simulink model "CLRFSPFCRealizedSimscape"  (R2025a)
settings: Solver=daessc  StartTime=0.0  StopTime=tend  FixedStep=tstep  MaxStep=1e-6  RelTol=1e-3  AbsTol=1e-4
undefined symbols (not defined in the file): Cf, fg, ncycles_end, Rc1, Rc2, Rc3, Rclp, Rin1, Rin2, Rin3, Rout, Rst1, Rst2, tend, Vc, Vg
libraries: fl_lib x48, nesl_utility x13, ee_lib x7, simulink x3, eePowerMeasurement x1, eeRmsMeasurement x1
settings Model: Creator=FactCore  LastModifiedBy=FactCore
settings SolverCC: ZeroCrossAlgorithm=Adaptive  SolverResetMethod=Robust
settings DataIOCC: SaveTime=off
settings HardwareCC: ProdHWDeviceType=AMD->x86-64 (Windows64)
settings SFSimCC: SimTargetLang=C++  SimDLTargetLibrary=mkl-dnn

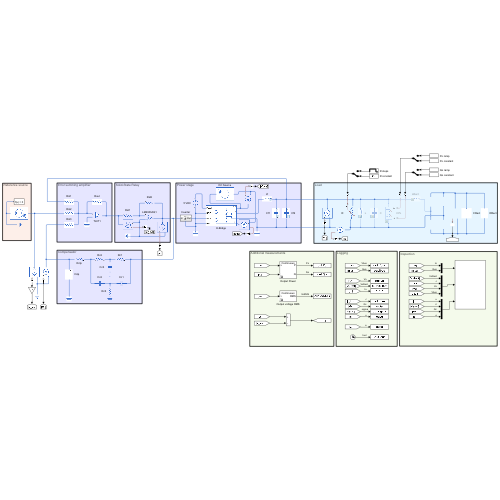
[thumbnail: Simulink's stored preview of the top-level diagram]
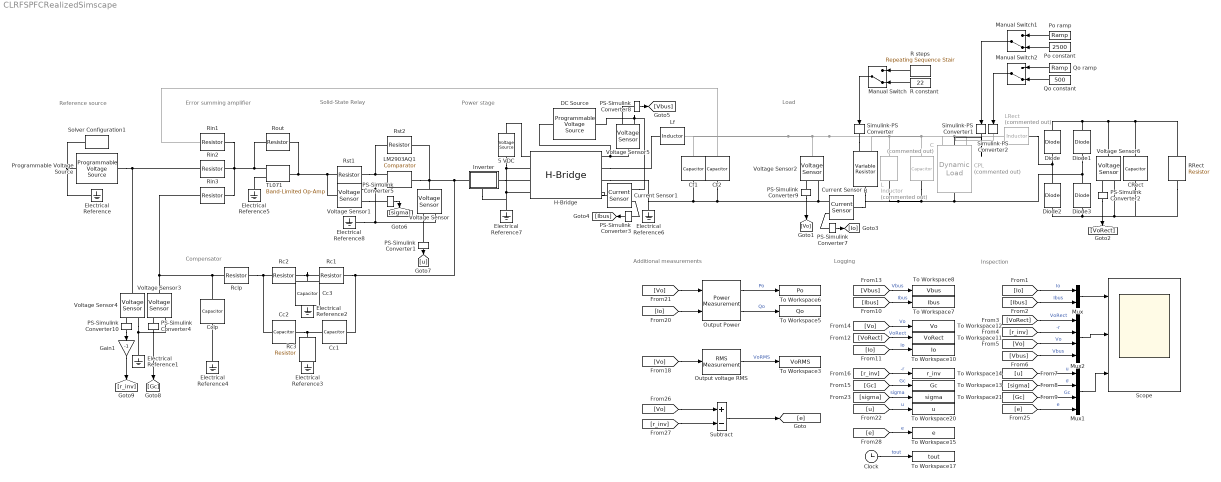
== system CLRFSPFCRealizedSimscape ==
  note: Additional measurements
  note: Inspection
  note: Logging
  note: Reference source
  note: Error summing amplifier
  note: Compensator
  note: Load
  note: Power stage
  note: Solid-State Relay
  5 VDC : ee_lib/Sources/Voltage Source  dc_voltage=5 V  ac_voltage=0 V  ac_shift=0 rad  ac_frequency=60 Hz  noise_mode=ee.enum.sources.noise.Disabled  PSD=0 V^2/Hz  sample_time=1e-3 s  repeatability=ee.enum.sources.repeatability.NotRepeatable  user_seed=0  auto_seed=3499211588  i_specify=off  i_priority=None  i=0 A  i_nominal_specify=off  i_nominal_value=1  i_nominal_unit=A  v_specify=off  v_priority=None  v=0 V  v_nominal_specify=off  v_nominal_value=1  v_nominal_unit=V
  C : fl_lib/Electrical/Electrical Elements/Capacitor  Commented=on  c=400e-6 F  r=1e-6 Ohm  g=0 1/Ohm  i_specify=off  i_priority=None  i=0 A  i_nominal_specify=off  i_nominal_value=1  i_nominal_unit=A  v_specify=off  v_priority=None  v=0 V  v_nominal_specify=off  v_nominal_value=1  v_nominal_unit=V  vc_specify=off  vc_priority=High  vc=0 V  vc_nominal_specify=off  vc_nominal_value=1  vc_nominal_unit=V
  CPL : ee_lib/Passive/Dynamic Load  Commented=on  load_type=ee.enum.dc_ac.ac  min_supply_voltage=20 V  pow_min=1e-3 W  G_reverse=1e-6 S  deltaV=1e-3 V  f0=fg Hz  Vrms_min=Vg/sqrt(2)*0.5 V  tau=0.01 s  Vrms_ini=Vg/sqrt(2) V  Vang_ini=0 deg
      settings: InternalSimscapePortConfiguration="{\"Bottom\":[],\"Left\":[{\"id\":\"p\",\"label\":\"+\",\"type\":\"foundation.electrical.electrical\"}],\"Right\":[{\"id\":\"n\",\"label\":\"-\",\"type\":\"foundation.electrical.electrical\"}],\"Top\":[{\"id\":\"P\",\"label\":\"P\",\"type\":\"input\"},{\"id\":\"Q\",\"label\":\"Q\",\"type\":\"input\"}]}"
  CRect : fl_lib/Electrical/Electrical Elements/Capacitor  c=100 uF  r=2 mOhm  g=0 1/Ohm  i_specify=off  i_priority=None  i=0 A  i_nominal_specify=off  i_nominal_value=1  i_nominal_unit=A  v_specify=off  v_priority=None  v=0 V  v_nominal_specify=off  v_nominal_value=1  v_nominal_unit=V  vc_specify=off  vc_priority=High  vc=0 V  vc_nominal_specify=off  vc_nominal_value=1  vc_nominal_unit=V
  Cc1 : fl_lib/Electrical/Electrical Elements/Capacitor  c=Cc1 F  r=1e-6 Ohm  g=0 1/Ohm  i_specify=off  i_priority=None  i=0 A  i_nominal_specify=off  i_nominal_value=1  i_nominal_unit=A  v_specify=off  v_priority=None  v=0 V  v_nominal_specify=off  v_nominal_value=1  v_nominal_unit=V  vc_specify=off  vc_priority=High  vc=0 V  vc_nominal_specify=off  vc_nominal_value=1  vc_nominal_unit=V
  Cc2 : fl_lib/Electrical/Electrical Elements/Capacitor  c=Cc2 F  r=1e-6 Ohm  g=0 1/Ohm  i_specify=off  i_priority=None  i=0 A  i_nominal_specify=off  i_nominal_value=1  i_nominal_unit=A  v_specify=off  v_priority=None  v=0 V  v_nominal_specify=off  v_nominal_value=1  v_nominal_unit=V  vc_specify=off  vc_priority=High  vc=0 V  vc_nominal_specify=off  vc_nominal_value=1  vc_nominal_unit=V
  Cc3 : fl_lib/Electrical/Electrical Elements/Capacitor  c=Cc3 F  r=1e-6 Ohm  g=0 1/Ohm  i_specify=off  i_priority=None  i=0 A  i_nominal_specify=off  i_nominal_value=1  i_nominal_unit=A  v_specify=off  v_priority=None  v=0 V  v_nominal_specify=off  v_nominal_value=1  v_nominal_unit=V  vc_specify=off  vc_priority=High  vc=0 V  vc_nominal_specify=off  vc_nominal_value=1  vc_nominal_unit=V
  Cclp : fl_lib/Electrical/Electrical Elements/Capacitor  c=Cclp F  r=1e-6 Ohm  g=0 1/Ohm  i_specify=off  i_priority=None  i=0 A  i_nominal_specify=off  i_nominal_value=1  i_nominal_unit=A  v_specify=off  v_priority=None  v=0 V  v_nominal_specify=off  v_nominal_value=1  v_nominal_unit=V  vc_specify=off  vc_priority=High  vc=0 V  vc_nominal_specify=off  vc_nominal_value=1  vc_nominal_unit=V
  Cf1 : fl_lib/Electrical/Electrical Elements/Capacitor  c=Cf/2 F  r=5e-3 Ohm  g=0 1/Ohm  i_specify=off  i_priority=None  i=0 A  i_nominal_specify=off  i_nominal_value=1  i_nominal_unit=A  v_specify=off  v_priority=None  v=0 V  v_nominal_specify=off  v_nominal_value=1  v_nominal_unit=V  vc_specify=off  vc_priority=High  vc=0 V  vc_nominal_specify=off  vc_nominal_value=1  vc_nominal_unit=V
  Cf2 : fl_lib/Electrical/Electrical Elements/Capacitor  c=Cf/2 F  r=5e-3 Ohm  g=0 1/Ohm  i_specify=off  i_priority=None  i=0 A  i_nominal_specify=off  i_nominal_value=1  i_nominal_unit=A  v_specify=off  v_priority=None  v=0 V  v_nominal_specify=off  v_nominal_value=1  v_nominal_unit=V  vc_specify=off  vc_priority=High  vc=0 V  vc_nominal_specify=off  vc_nominal_value=1  vc_nominal_unit=V
  Clock : Clock
  Current Sensor : fl_lib/Electrical/Electrical Sensors/Current Sensor
  Current Sensor1 : fl_lib/Electrical/Electrical Sensors/Current Sensor
  DC Source : ee_lib/Sources/Programmable Voltage Source  magnitude_type=ee.enum.timechanging.constant  ac_magnitude=0 V  magn_ramp=1 V/s  magn_step=40*sqrt(2) V  magn_modu_magn=1 V  magn_modu_freq=1 Hz  magn_t1=tend-9/(4*fg) s  magn_t2=tend-3/(4*fg) s  frequency_type=ee.enum.timechanging.constant  ac_frequency=fg*10 Hz  freq_ramp=1 Hz/s  freq_step=1 Hz  freq_modu_magn=1 Hz  freq_modu_freq=1 Hz  freq_t1=1 s  freq_t2=2 s  phase_type=ee.enum.timechanging.constant  ac_shift=0 deg  phase_ramp=1 deg/s  phase_step=1 deg  phase_modu_magn=1 deg  phase_modu_freq=1 Hz  phase_t1=1 s  phase_t2=2 s  dc_type=ee.enum.timechanging.constant  dc_voltage=E V  dc_ramp=1 V/s  dc_step=E*3/8 V  dc_modu_magn=1 V  dc_modu_freq=1 Hz  dc_t1=tend-9/(4*fg) s  dc_t2=tend-3/(4*fg) s  harmonic_option=0  harmonic_orders=[5, 7, 11, 13]  harmonic_ratios=[.1, .1, .1, .1]  harmonic_shifts=[0, 0, 0, 0] deg  harmonic_t1=-inf s  harmonic_t2=inf s  noise_mode=0  PSD=0 V^2/Hz  repeatability=1  auto_seed=0  user_seed=0  sample_time=1e-3 s  i_specify=off  i_priority=None  i=0 A  i_nominal_specify=off  i_nominal_value=1  i_nominal_unit=A  v_specify=off  v_priority=None  v=0 V  v_nominal_specify=off  v_nominal_value=1  v_nominal_unit=V
      settings: InternalSimscapePortConfiguration="{\"Bottom\":[],\"Left\":[{\"id\":\"p\",\"label\":\"+\",\"type\":\"foundation.electrical.electrical\"}],\"Right\":[{\"id\":\"n\",\"label\":\"-\",\"type\":\"foundation.electrical.electrical\"}],\"Top\":[]}"
  Diode{,1..3} (4 alike) : fl_lib/Electrical/Electrical Elements/Diode  Vf=0.6 V  Ron=0.3 Ohm  Goff=1e-8 1/Ohm  i_specify=off  i_priority=None  i=0 A  i_nominal_specify=off  i_nominal_value=1  i_nominal_unit=A  v_specify=off  v_priority=None  v=0 V  v_nominal_specify=off  v_nominal_value=1  v_nominal_unit=V
  Electrical Reference{,1..8} (9 alike) : fl_lib/Electrical/Electrical Elements/Electrical Reference
  Gain1 : Gain  Gain=-1
  H-Bridge : ee_lib/Semiconductors & Converters/Converters/H-Bridge  supply_ports=ee.enum.supply_ports.showsupply  pwm_or_av=ee.enum.pwm_or_av.pwm  regenerative_braking_mode=ee.enum.converters.regenerative_braking_mode.depends_on_rev  discontinuous=ee.enum.current_profile.continuous  freewheeling_mode=ee.enum.converters.freewheeling_mode.two_diodes  Rload=10 Ohm  Lload=1e-5 H  F=10 kHz  Venable=2.5 V  Vmax=5.0 V  Vreverse=0.1 V  Vbrake=2.5 V  Vm=12 V  Ron=0.1 Ohm  Don=0.05 Ohm  Goff=1e-6 S  Tmeas=298.15 K  Ron2=0.1 Ohm  Don2=0.05 Ohm  Tmeas2=398.15 K  thermal_mass=100 J/K  initial_temperature=298.15 K
      settings: InternalSimscapePortConfiguration="{\"Bottom\":[],\"Left\":[{\"id\":\"ENA\",\"label\":\"PWM\",\"type\":\"foundation.electrical.electrical\"},{\"id\":\"REF\",\"label\":\"REF\",\"type\":\"foundation.electrical.electrical\"},{\"id\":\"REV\",\"label\":\"REV\",\"type\":\"foundation.electrical.electrical\"},{\"id\":\"BRK\",\"label\":\"BRK\",\"type\":\"foundation.electrical.electrical\"}],\"Right\":[{\"id\":\"p1\",\"label\":\"V+\",\"type\":\"foundation.electrical.electrical\"},{\"id\":\"p2\",\"label\":\"+\",\"type\":\"foundation.electrical.electrical\"},{\"id\":\"n2\",\"label\":\"-\",\"type\":\"foundation.electrical.electrical\"},{\"id\":\"n1\",\"label\":\"V-\",\"type\":\"foundation.electrical.electrical\"}],\"Top\":[]}"
  Inverter : Subsystem
      settings: PortSchema="{\"entries\":[{\"content\":{\"sides\":[{\"content\":{\"connectorIds\":[\"LConn1\"]},\"type\":\"ConnectorPlacement.EquallySpacedRectSide\",\"uuid\":\"424ab37e-a00b-460f-b115-faa5b36651fc\"},{\"content\":{\"connectorIds\":[\"RConn1\"],\"side\":\"RIGHT\"},\"type\":\"ConnectorPlacement.EquallySpacedRectSide\",\"uuid\":\"a9dc5729-7781-4560-822f-9114a4c128a2\"},{\"content\":{\"side\":\"TOP\"},\"type\":\"ConnectorPlacement.EquallySpacedRectSide\",\"uuid\":\"cc59a33d-4be6-4989-bd27-692f8e76c2fa\"},{\"content\":{\"connectorIds\":[\"RConn2\"],\"side\":\"BOTTOM\"},\"type\":\"ConnectorPlacement.EquallySpacedRectSide\",\"uuid\":\"b5b66fbd-1a2c-4a2d-a2ac-28cbb2475c69\"}]},\"type\":\"ConnectorPlacement.EquallySpacedConnector\",\"uuid\":\"de6c9a9d-c841-40e7-b68c-d24e9f712a00\"}],\"packageUris\":[\"http://schema.mathworks.com/mf0/Connector/R2020b\"],\"version\":\"1.0\"}"
  L : fl_lib/Electrical/Electrical Elements/Inductor  Commented=on  l=400 mH  r=1 Ohm  g=1e-9 1/Ohm  i_specify=off  i_priority=None  i=0 A  i_nominal_specify=off  i_nominal_value=1  i_nominal_unit=A  v_specify=off  v_priority=None  v=0 V  v_nominal_specify=off  v_nominal_value=1  v_nominal_unit=V  i_L_specify=off  i_L_priority=High  i_L=0 A  i_L_nominal_specify=off  i_L_nominal_value=1  i_L_nominal_unit=A
  LM2903AQ1 : ee_lib/Integrated Circuits/Comparator  V_OS=1 mV  C_IN=0 pF  V_OL=-Vc V  V_OH=Vc V  R_OUT=50 Ohm  Delay=1.3 us
      settings: InternalSimscapePortConfiguration="{\"Bottom\":[],\"Left\":[{\"id\":\"p\",\"label\":\"+\",\"type\":\"foundation.electrical.electrical\"},{\"id\":\"n\",\"label\":\"-\",\"type\":\"foundation.electrical.electrical\"}],\"Right\":[{\"id\":\"J\",\"label\":\"\",\"type\":\"foundation.electrical.electrical\"}],\"Top\":[]}"
  LRect : fl_lib/Electrical/Electrical Elements/Inductor  Commented=on  l=22 uH  r=1 mOhm  g=1e-9 1/Ohm  i_specify=off  i_priority=None  i=0 A  i_nominal_specify=off  i_nominal_value=1  i_nominal_unit=A  v_specify=off  v_priority=None  v=0 V  v_nominal_specify=off  v_nominal_value=1  v_nominal_unit=V  i_L_specify=off  i_L_priority=High  i_L=0 A  i_L_nominal_specify=off  i_L_nominal_value=1  i_L_nominal_unit=A
  Lf : fl_lib/Electrical/Electrical Elements/Inductor  l=Lf H  r=Rf Ohm  g=1e-9 1/Ohm  i_specify=off  i_priority=None  i=0 A  i_nominal_specify=off  i_nominal_value=1  i_nominal_unit=A  v_specify=off  v_priority=None  v=0 V  v_nominal_specify=off  v_nominal_value=1  v_nominal_unit=V  i_L_specify=off  i_L_priority=High  i_L=0 A  i_L_nominal_specify=off  i_L_nominal_value=1  i_L_nominal_unit=A
  Manual Switch : ManualSwitch  CurrentSetting=0
  Manual Switch1 : ManualSwitch  CurrentSetting=0
  Manual Switch2 : ManualSwitch  CurrentSetting=0
  Mux : Mux  Inputs=2
  Mux1 : Mux
  Mux2 : Mux
  Output Power : eePowerMeasurement/Power Measurement  LabelModeActiveChoice=Continuous  F=fg  K=[1]  Ts=0
  Output voltage RMS : eeRmsMeasurement/RMS Measurement  LabelModeActiveChoice=Total  F=fg  SpecifyHarmonics=off  K=[0 1 2]  Ts=0
      settings: LibrarySourceBlock=|
      | ee_sl_lib/Measurements/RMS
      | Measurement
  PS-Simulink Converter{1..5,7..10} (9 alike) : nesl_utility/PS-Simulink Converter  PhysicalDomain=network_engine_domain  SubClassName=ps_output  LeftPortType=input  RightPortType=output  PseudoPeriodic=off  Frequencies=[]  VectorFormat=inherit  Unit=inherit  AffineConversion=off
  Po constant : Constant  Value=2500
  Po ramp : simulink/Sources/Ramp  slope=5000*fg/(ncycles_end-2)  start=2/fg  InitialOutput=0
  Programmable Voltage Source : ee_lib/Sources/Programmable Voltage Source  magnitude_type=ee.enum.timechanging.constant  ac_magnitude=Vg V  magn_ramp=Vg*fg/(ncycles_end) V/s  magn_step=-Vg/2 V  magn_modu_magn=1 V  magn_modu_freq=1 Hz  magn_t1=tend-9/(4*fg) s  magn_t2=tend-3/(4*fg) s  frequency_type=ee.enum.timechanging.constant  ac_frequency=fg Hz  freq_ramp=1 Hz/s  freq_step=1 Hz  freq_modu_magn=1 Hz  freq_modu_freq=1 Hz  freq_t1=1 s  freq_t2=2 s  phase_type=ee.enum.timechanging.constant  ac_shift=0 deg  phase_ramp=1 deg/s  phase_step=180 deg  phase_modu_magn=1 deg  phase_modu_freq=1 Hz  phase_t1=tend-8/(4*fg) s  phase_t2=tend-3/(4*fg) s  dc_type=ee.enum.timechanging.constant  dc_voltage=0 V  dc_ramp=1 V/s  dc_step=1 V  dc_modu_magn=1 V  dc_modu_freq=1 Hz  dc_t1=1 s  dc_t2=2 s  harmonic_option=0  harmonic_orders=[5, 7, 11, 13]  harmonic_ratios=[.1, .1, .1, .1]  harmonic_shifts=[0, 0, 0, 0] deg  harmonic_t1=-inf s  harmonic_t2=inf s  noise_mode=0  PSD=0 V^2/Hz  repeatability=1  auto_seed=0  user_seed=0  sample_time=1e-3 s  i_specify=off  i_priority=None  i=0 A  i_nominal_specify=off  i_nominal_value=1  i_nominal_unit=A  v_specify=off  v_priority=None  v=0 V  v_nominal_specify=off  v_nominal_value=1  v_nominal_unit=V
      settings: InternalSimscapePortConfiguration="{\"Bottom\":[],\"Left\":[{\"id\":\"p\",\"label\":\"+\",\"type\":\"foundation.electrical.electrical\"}],\"Right\":[{\"id\":\"n\",\"label\":\"-\",\"type\":\"foundation.electrical.electrical\"}],\"Top\":[]}"
  Qo constant : Constant  Value=500
  Qo ramp : simulink/Sources/Ramp  slope=5000*fg/(ncycles_end-2)  start=2/fg  InitialOutput=0
  R : fl_lib/Electrical/Electrical Elements/Variable Resistor  Rmin=0 Ohm  thermalEnable=false  thermal_mass=1 J/K  i_specify=off  i_priority=None  i=0 A  i_nominal_specify=off  i_nominal_value=1  i_nominal_unit=A  v_specify=off  v_priority=None  v=0 V  v_nominal_specify=off  v_nominal_value=1  v_nominal_unit=V  T_specify=off  T_priority=None  T=300 K  T_nominal_specify=off  T_nominal_value=1  T_nominal_unit=K
  R constant : Constant  Value=22
  R steps : simulink/Sources/Repeating Sequence Stair  OutValues=[repmat(1e4, 1, ncycles_end-2), 22, 11]  tsamp=1/fg  OutMin=[]  OutMax=[]  OutDataTypeStr=double  OutputDataTypeScalingMode=double  OutDataType=fixdt(0,8)  ConRadixGroup=Best Precision: Vector-wise  OutScaling=2^-12
  RRect : fl_lib/Electrical/Electrical Elements/Resistor  R=22 Ohm  i_specify=off  i_priority=None  i=0 A  i_nominal_specify=off  i_nominal_value=1  i_nominal_unit=A  v_specify=off  v_priority=None  v=0 V  v_nominal_specify=off  v_nominal_value=1  v_nominal_unit=V
  Rc1 : fl_lib/Electrical/Electrical Elements/Resistor  R=Rc1 Ohm  i_specify=off  i_priority=None  i=0 A  i_nominal_specify=off  i_nominal_value=1  i_nominal_unit=A  v_specify=off  v_priority=None  v=0 V  v_nominal_specify=off  v_nominal_value=1  v_nominal_unit=V
  Rc2 : fl_lib/Electrical/Electrical Elements/Resistor  R=Rc2 Ohm  i_specify=off  i_priority=None  i=0 A  i_nominal_specify=off  i_nominal_value=1  i_nominal_unit=A  v_specify=off  v_priority=None  v=0 V  v_nominal_specify=off  v_nominal_value=1  v_nominal_unit=V
  Rc3 : fl_lib/Electrical/Electrical Elements/Resistor  R=Rc3 Ohm  i_specify=off  i_priority=None  i=0 A  i_nominal_specify=off  i_nominal_value=1  i_nominal_unit=A  v_specify=off  v_priority=None  v=0 V  v_nominal_specify=off  v_nominal_value=1  v_nominal_unit=V
  Rclp : fl_lib/Electrical/Electrical Elements/Resistor  R=Rclp Ohm  i_specify=off  i_priority=None  i=0 A  i_nominal_specify=off  i_nominal_value=1  i_nominal_unit=A  v_specify=off  v_priority=None  v=0 V  v_nominal_specify=off  v_nominal_value=1  v_nominal_unit=V
  Rin1 : fl_lib/Electrical/Electrical Elements/Resistor  R=Rin1 Ohm  i_specify=off  i_priority=None  i=0 A  i_nominal_specify=off  i_nominal_value=1  i_nominal_unit=A  v_specify=off  v_priority=None  v=0 V  v_nominal_specify=off  v_nominal_value=1  v_nominal_unit=V
  Rin2 : fl_lib/Electrical/Electrical Elements/Resistor  R=Rin2 Ohm  i_specify=off  i_priority=None  i=0 A  i_nominal_specify=off  i_nominal_value=1  i_nominal_unit=A  v_specify=off  v_priority=None  v=0 V  v_nominal_specify=off  v_nominal_value=1  v_nominal_unit=V
  Rin3 : fl_lib/Electrical/Electrical Elements/Resistor  R=Rin3 Ohm  i_specify=off  i_priority=None  i=0 A  i_nominal_specify=off  i_nominal_value=1  i_nominal_unit=A  v_specify=off  v_priority=None  v=0 V  v_nominal_specify=off  v_nominal_value=1  v_nominal_unit=V
  Rout : fl_lib/Electrical/Electrical Elements/Resistor  R=Rout Ohm  i_specify=off  i_priority=None  i=0 A  i_nominal_specify=off  i_nominal_value=1  i_nominal_unit=A  v_specify=off  v_priority=None  v=0 V  v_nominal_specify=off  v_nominal_value=1  v_nominal_unit=V
  Rst1 : fl_lib/Electrical/Electrical Elements/Resistor  R=Rst1 Ohm  i_specify=off  i_priority=None  i=0 A  i_nominal_specify=off  i_nominal_value=1  i_nominal_unit=A  v_specify=off  v_priority=None  v=0 V  v_nominal_specify=off  v_nominal_value=1  v_nominal_unit=V
  Rst2 : fl_lib/Electrical/Electrical Elements/Resistor  R=Rst2 Ohm  i_specify=off  i_priority=None  i=0 A  i_nominal_specify=off  i_nominal_value=1  i_nominal_unit=A  v_specify=off  v_priority=None  v=0 V  v_nominal_specify=off  v_nominal_value=1  v_nominal_unit=V
  Scope : Scope  NumInputPorts=3
      settings: ActiveDisplayYMinimum=-37.238924099797785  ActiveDisplayYMaximum=37.232975162618189
  Simulink-PS Converter : nesl_utility/Simulink-PS Converter  PhysicalDomain=network_engine_domain  SubClassName=ps_input  LeftPortType=input  RightPortType=output  PseudoPeriodic=off  Frequencies=[]  NoiseDistribution=none  NoiseParameters=[]  Unit=1  AffineConversion=off  FilteringAndDerivatives=provide  SimscapeFilterOrder=1  InputFilterTimeConstant=0.001  UdotUserProvided=0
  Simulink-PS Converter1 : nesl_utility/Simulink-PS Converter  PhysicalDomain=network_engine_domain  SubClassName=ps_input  LeftPortType=input  RightPortType=output  PseudoPeriodic=off  Frequencies=[]  NoiseDistribution=none  NoiseParameters=[]  Unit=1  AffineConversion=off  FilteringAndDerivatives=provide  SimscapeFilterOrder=1  InputFilterTimeConstant=0.001  UdotUserProvided=0
  Simulink-PS Converter2 : nesl_utility/Simulink-PS Converter  PhysicalDomain=network_engine_domain  SubClassName=ps_input  LeftPortType=input  RightPortType=output  PseudoPeriodic=off  Frequencies=[]  NoiseDistribution=none  NoiseParameters=[]  Unit=1  AffineConversion=off  FilteringAndDerivatives=provide  SimscapeFilterOrder=1  InputFilterTimeConstant=0.001  UdotUserProvided=0
  Solver Configuration1 : nesl_utility/Solver Configuration  PhysicalDomain=network_engine_domain  SubClassName=solver  LeftPortType=input  RightPortType=generic  Tones=[]  Harmonics=[]  SimulateNoise=off  Profile=off  UseLocalSampling=off  EnableSwitchedLinearOptims=on  FrequencyDomain=off  UseCCode=off  RelTol=0.001  AbsTol=0.001  MinStep=1e-09  ToWorkspace=off  RevertToSquareIcSolve=off  NumHomotopyIterations=100  PhasorMode=off  PhasorModeNumHarmonics=1  ConsistencySolver=NEWTON_XTOL_AFTER_FTOL  IndexReductionMethod=DerivativeReplacement  DoDC=off  ResidualTolerance=1e-09  ConsistencyTolSource=GLOBAL  ConsistencyAbsTol=0.001  ConsistencyRelTol=0.001  ConsistencyTolFactor=0.001  UseLocalSolver=off  LocalSolverChoice=NE_BACKWARD_EULER_ADVANCER  ResolveIndetEquations=on  FunctionEvalNumThread=1  LocalSolverSampleTime=0.001  DoFixedCost=off  MaxNonlinIter=3  MaxModeIter=2  ComputeImpulses=off  ImpulseIterations=2  LinearAlgebra=auto  LinearAlgebraNumThread=0  EquationFormulation=NE_TIME_EF  DelaysMemoryBudget=4096  AutomaticFiltering=on  FilteringTimeConstant=0.001  PartitionStorageMethod=AS_NEEDED  PartitionMemoryBudget=1024  PartitionMethod=ROBUST  MultibodyUseLocalSolver=off  MultibodyLocalSolverChoice=ODE1  MultibodyLocalSolverSampleTime=0.001
  Subtract : Sum  Inputs=+-
  TL071 : ee_lib/Integrated Circuits/Band-Limited Op-Amp  A=200000  Rin=1e6 Ohm  Rout=0.3 Ohm  Vmin=-Vc V  Vmax=Vc V  Vdotmax=20000000 V/s  f=1e6 Hz  V0=1 mV
  To Workspace10 : ToWorkspace  VariableName=Io  SampleTime=-1
      settings: Decimation=outDec
  To Workspace11 : ToWorkspace  VariableName=VoRect  SampleTime=-1
      settings: Decimation=outDec
  To Workspace12 : ToWorkspace  VariableName=Vo  SampleTime=-1
      settings: Decimation=outDec
  To Workspace13 : ToWorkspace  VariableName=Gc  SampleTime=-1
      settings: Decimation=outDec
  To Workspace14 : ToWorkspace  VariableName=r_inv  SampleTime=-1
      settings: Decimation=outDec
  To Workspace15 : ToWorkspace  VariableName=e  SampleTime=-1
      settings: Decimation=outDec
  To Workspace17 : ToWorkspace  VariableName=tout  SampleTime=-1
      settings: Decimation=outDec
  To Workspace20 : ToWorkspace  VariableName=u  SampleTime=-1
      settings: Decimation=outDec
  To Workspace21 : ToWorkspace  VariableName=sigma  SampleTime=-1
      settings: Decimation=outDec
  To Workspace3 : ToWorkspace  VariableName=VoRMS  SampleTime=-1
      settings: Decimation=outDec
  To Workspace5 : ToWorkspace  VariableName=Qo  SampleTime=-1
      settings: Decimation=outDec
  To Workspace6 : ToWorkspace  VariableName=Po  SampleTime=-1
      settings: Decimation=outDec
  To Workspace7 : ToWorkspace  VariableName=Ibus  SampleTime=-1
      settings: Decimation=outDec
  To Workspace8 : ToWorkspace  VariableName=Vbus  SampleTime=-1
      settings: Decimation=outDec
  Voltage Sensor{,1..6} (7 alike) : fl_lib/Electrical/Electrical Sensors/Voltage Sensor
  wires:
  [VoRect] -> Mux2/1  "VoRect"
  [Io] -> Mux/1  "Io"
  [Vo] -> Mux2/3  "Vo"
  [u] -> Mux1/1  "u"
  [sigma] -> Mux1/2  "σ"
  [r_inv] -> Mux2/2  "-r"
  [Gc] -> Mux1/3  "Gc"
  Mux1/1 -> Scope/3
  [Vbus] -> Mux2/4  "Vbus"
  Mux/1 -> Scope/1
  [Ibus] -> Mux/2  "Ibus"
  Mux2/1 -> Scope/2
  Manual Switch/1 -> Simulink-PS Converter/1
  R steps/1 -> Manual Switch/1
  R constant/1 -> Manual Switch/2
  PS-Simulink Converter9/1 -> [Vo]
  PS-Simulink Converter2/1 -> [VoRect]
  PS-Simulink Converter7/1 -> [Io]
  PS-Simulink Converter3/1 -> [Ibus]
  PS-Simulink Converter8/1 -> [Vbus]
  PS-Simulink Converter5/1 -> [sigma]
  PS-Simulink Converter1/1 -> [u]
  PS-Simulink Converter4/1 -> [Gc]
  PS-Simulink Converter10/1 -> Gain1/1
  Gain1/1 -> [r_inv]
  [Vbus] -> To Workspace8/1  "Vbus"
  [Ibus] -> To Workspace7/1  "Ibus"
  [Io] -> To Workspace10/1  "Io"
  [VoRect] -> To Workspace11/1  "VoRect"
  [Vo] -> To Workspace12/1  "Vo"
  [Gc] -> To Workspace13/1  "Gc"
  [r_inv] -> To Workspace14/1  "-r"
  [u] -> To Workspace20/1  "u"
  [sigma] -> To Workspace21/1  "sigma"
  [Vo] -> Output Power/1
  [Io] -> Output Power/2
  Output Power/2 -> To Workspace5/1  "Qo"
  Output Power/1 -> To Workspace6/1  "Po"
  [Vo] -> Output voltage RMS/1
  Output voltage RMS/1 -> To Workspace3/1  "VoRMS"
  [e] -> Mux1/4  "e"
  [Vo] -> Subtract/1
  [r_inv] -> Subtract/2
  Subtract/1 -> [e]
  Clock/1 -> To Workspace17/1  "tout"
  [e] -> To Workspace15/1  "e"
  Po constant/1 -> Manual Switch1/2
  Manual Switch1/1 -> Simulink-PS Converter1/1
  Po ramp/1 -> Manual Switch1/1
  Qo ramp/1 -> Manual Switch2/1
  Qo constant/1 -> Manual Switch2/2
  Manual Switch2/1 -> Simulink-PS Converter2/1
  connections:
  Rst1/RConn1 -- LM2903AQ1/LConn1 -- Rst2/LConn1
  Solver Configuration1/RConn1 -- Electrical Reference/LConn1 -- Programmable Voltage Source/RConn1
  Electrical Reference2/LConn1 -- Cc3/RConn1
  Electrical Reference3/LConn1 -- Rc3/RConn1
  H-Bridge/RConn1 -- DC Source/LConn1 -- Voltage Sensor5/LConn1
  Voltage Sensor5/RConn2 -- Current Sensor1/RConn2 -- DC Source/RConn1
  Rc2/LConn1 -- Cc3/LConn1 -- Rc1/RConn1
  Cc1/RConn1 -- Cc2/LConn1 -- Rc3/LConn1
  Cc2/RConn1 -- Rclp/LConn1 -- Rc2/RConn1
  Voltage Sensor3/LConn1 -- Rin3/LConn1 -- Cclp/LConn1 -- Rclp/RConn1
  Voltage Sensor4/RConn2 -- Electrical Reference1/LConn1 -- Voltage Sensor3/RConn2
  Voltage Sensor/RConn2 -- LM2903AQ1/LConn2 -- Voltage Sensor1/RConn2 -- Electrical Reference8/LConn1
  Rin2/RConn1 -- Rin3/RConn1 -- Rin1/RConn1 -- TL071/LConn2 -- Rout/LConn1
  Diode1/LConn1 -- CPL/RConn1 -- R/RConn1 -- Current Sensor/LConn1 -- L/RConn1 -- C/RConn1 -- Diode3/RConn1
  TL071/LConn1 -- Electrical Reference5/LConn1
  Rout/RConn1 -- TL071/RConn1 -- Voltage Sensor1/LConn1 -- Rst1/LConn1
  Rc1/LConn1 -- Inverter/LConn1 -- LM2903AQ1/RConn1 -- Voltage Sensor/LConn1 -- Rst2/RConn1 -- Cc1/LConn1
  H-Bridge/RConn2 -- Lf/LConn1
  Voltage Sensor4/LConn1 -- Programmable Voltage Source/LConn1 -- Rin2/LConn1
  H-Bridge/LConn2 -- 5 VDC/RConn1 -- Inverter/RConn2 -- Electrical Reference7/LConn1 -- H-Bridge/LConn4
  Current Sensor/RConn2 -- Cf2/RConn1 -- Cf1/RConn1 -- H-Bridge/RConn3 -- Electrical Reference6/LConn1 -- Voltage Sensor2/RConn2
  Diode2/LConn1 -- RRect/RConn1 -- CRect/RConn1 -- Voltage Sensor6/RConn2 -- Diode3/LConn1
  C/LConn1 -- CPL/LConn1 -- LRect/LConn1 -- L/LConn1 -- Cf1/LConn1 -- Lf/RConn1 -- Rin1/LConn1 -- Cf2/LConn1 -- Voltage Sensor2/LConn1 -- R/LConn2
  Electrical Reference4/LConn1 -- Cclp/RConn1
  5 VDC/LConn1 -- H-Bridge/LConn1
  CRect/LConn1 -- Diode/RConn1 -- Diode1/RConn1 -- Voltage Sensor6/LConn1 -- RRect/LConn1
  Diode/LConn1 -- Diode2/RConn1 -- LRect/RConn1
  Current Sensor1/LConn1 -- H-Bridge/RConn4
  Inverter/RConn1 -- H-Bridge/LConn3
  Simulink-PS Converter/RConn1 -- R/LConn1
  PS-Simulink Converter9/LConn1 -- Voltage Sensor2/RConn1
  PS-Simulink Converter2/LConn1 -- Voltage Sensor6/RConn1
  PS-Simulink Converter7/LConn1 -- Current Sensor/RConn1
  PS-Simulink Converter3/LConn1 -- Current Sensor1/RConn1
  PS-Simulink Converter8/LConn1 -- Voltage Sensor5/RConn1
  Voltage Sensor1/RConn1 -- PS-Simulink Converter5/LConn1
  PS-Simulink Converter1/LConn1 -- Voltage Sensor/RConn1
  PS-Simulink Converter4/LConn1 -- Voltage Sensor3/RConn1
  PS-Simulink Converter10/LConn1 -- Voltage Sensor4/RConn1
  Simulink-PS Converter1/RConn1 -- CPL/LConn2
  CPL/LConn3 -- Simulink-PS Converter2/RConn1

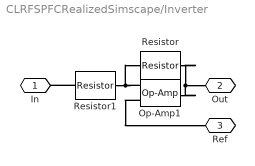
== system CLRFSPFCRealizedSimscape/Inverter ==
  Op-Amp1 : fl_lib/Electrical/Electrical Elements/Op-Amp  outI_specify=off  outI_priority=None  outI=0 A  outI_nominal_specify=off  outI_nominal_value=1  outI_nominal_unit=A
  Resistor : fl_lib/Electrical/Electrical Elements/Resistor  R=10e3 Ohm  i_specify=off  i_priority=None  i=0 A  i_nominal_specify=off  i_nominal_value=1  i_nominal_unit=A  v_specify=off  v_priority=None  v=0 V  v_nominal_specify=off  v_nominal_value=1  v_nominal_unit=V
  Resistor1 : fl_lib/Electrical/Electrical Elements/Resistor  R=10e3 Ohm  i_specify=off  i_priority=None  i=0 A  i_nominal_specify=off  i_nominal_value=1  i_nominal_unit=A  v_specify=off  v_priority=None  v=0 V  v_nominal_specify=off  v_nominal_value=1  v_nominal_unit=V
  In : PMIOPort  Side=Left
  Out : PMIOPort  Port=2  Side=Right
  Ref : PMIOPort  Port=3  Side=Right
  connections:
  Resistor/RConn1 -- Out/RConn1 -- Op-Amp1/RConn1
  Resistor1/LConn1 -- In/RConn1
  Resistor1/RConn1 -- Op-Amp1/LConn2 -- Resistor/LConn1
  Op-Amp1/LConn1 -- Ref/RConn1
